simulink subsystem "FuelCellCore"  (R2025b)
settings: Solver=VariableStepAuto  StartTime=0.0  StopTime=10.0  RelTol=1e-3
undefined symbols (not defined in the file): PlntFcAuxPwrMap, PlntFcCurrBpt, PlntFcH2FlwMap, PlntFcHeatFlwMap, PlntFcTempBpt, PlntFcVoltageMap
settings Model: ModifiedByFormat=The MathWorks, Inc.  Creator=The MathWorks, Inc.  LastModifiedBy=The MathWorks, Inc.
settings SolverCC: MaxZcPerStep=1.0
settings OptimizationCC: ReuseModelBlockBuffer=off
settings DebuggingCC: UnconnectedInputMsg=warning  UnconnectedOutputMsg=warning  UnconnectedLineMsg=warning  SubsystemReferenceDiagnosticForUnitTest=warning
settings ModelReferenceCC: EnableRefExpFcnMdlSchedulingChecks=on
settings RTWCC: GPUComputeCapability=3.5  DLArmComputeVersion=19.05

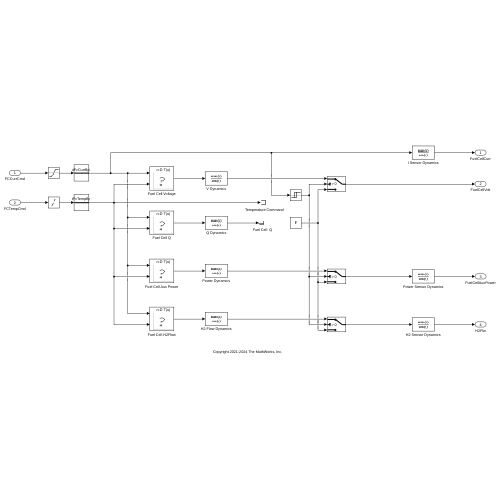
[thumbnail: Simulink's stored preview of the top-level diagram]
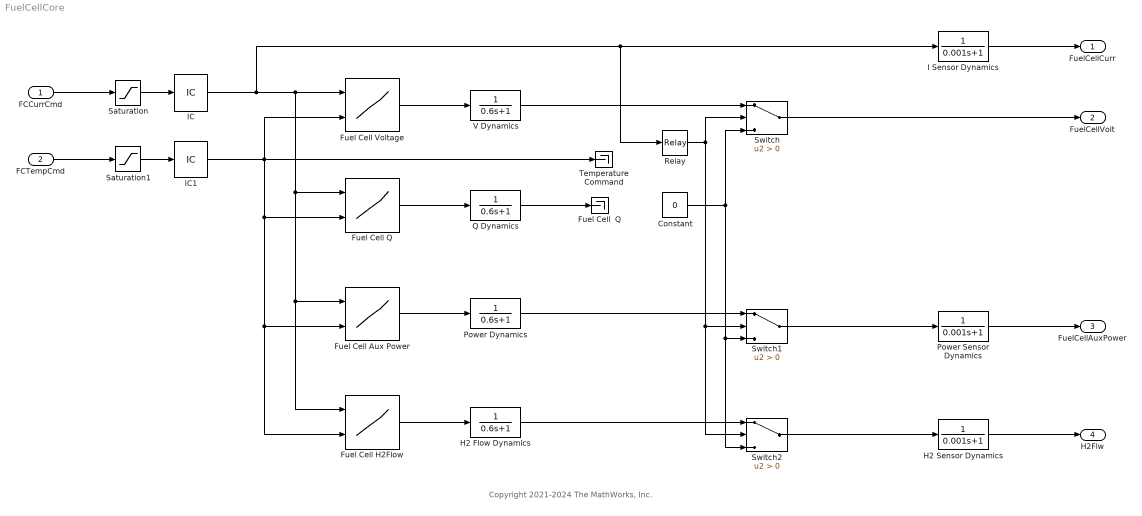
== system FuelCellCore ==
  note: Copyright 2021-2024 The MathWorks, Inc.
  FCCurrCmd : Inport
  FCTempCmd : Inport  Port=2
  Constant : Constant  Value=0
  Fuel Cell  Q : Terminator
  Fuel Cell Aux Power : Lookup_n-D  BreakpointsForDimension1=PlntFcCurrBpt  BreakpointsForDimension2=PlntFcTempBpt  Table=PlntFcAuxPwrMap  ExtrapMethod=Clip  InternalRulePriority=Speed  RndMeth=Simplest
      settings: InputPortMap=u0,u1
  Fuel Cell H2Flow : Lookup_n-D  BreakpointsForDimension1=PlntFcCurrBpt  BreakpointsForDimension2=PlntFcTempBpt  Table=PlntFcH2FlwMap  ExtrapMethod=Clip  InternalRulePriority=Speed  RndMeth=Simplest
      settings: InputPortMap=u0,u1
  Fuel Cell Q : Lookup_n-D  BreakpointsForDimension1=PlntFcCurrBpt  BreakpointsForDimension2=PlntFcTempBpt  Table=PlntFcHeatFlwMap  ExtrapMethod=Clip  InternalRulePriority=Speed  RndMeth=Simplest
      settings: InputPortMap=u0,u1
  Fuel Cell Voltage : Lookup_n-D  BreakpointsForDimension1=PlntFcCurrBpt  BreakpointsForDimension2=PlntFcTempBpt  Table=PlntFcVoltageMap  ExtrapMethod=Clip  InternalRulePriority=Speed  RndMeth=Simplest
      settings: InputPortMap=u0,u1
  H2 Flow Dynamics : TransferFcn  Denominator=[0.6 1]
  H2 Sensor Dynamics : TransferFcn  Denominator=[0.001 1]
  I Sensor Dynamics : TransferFcn  Denominator=[0.001 1]
  IC : InitialCondition  Value=PlntFcCurrBpt(1)
  IC1 : InitialCondition  Value=PlntFcTempBpt(1)
  Power Dynamics : TransferFcn  Denominator=[0.6 1]
  Power Sensor Dynamics : TransferFcn  Denominator=[0.001 1]
  Q Dynamics : TransferFcn  Denominator=[0.6 1]
  Relay : Relay
  Saturation : Saturate  UpperLimit=max(PlntFcCurrBpt)  LowerLimit=0  ZeroCross=off
  Saturation1 : Saturate  UpperLimit=max(PlntFcTempBpt)  LowerLimit=0  ZeroCross=off
  Switch : Switch  Criteria=u2 > Threshold  ZeroCross=off  SaturateOnIntegerOverflow=off  InputSameDT=off
  Switch1 : Switch  Criteria=u2 > Threshold  ZeroCross=off  SaturateOnIntegerOverflow=off  InputSameDT=off
  Switch2 : Switch  Criteria=u2 > Threshold  ZeroCross=off  SaturateOnIntegerOverflow=off  InputSameDT=off
  Temperature Command : Terminator
  V Dynamics : TransferFcn  Denominator=[0.6 1]
  FuelCellCurr : Outport
  FuelCellVolt : Outport  Port=2
  FuelCellAuxPower : Outport  Port=3
  H2Flw : Outport  Port=4
  wires:
  Q Dynamics/1 -> Fuel Cell  Q/1
  Saturation1/1 -> IC1/1
  H2 Sensor Dynamics/1 -> H2Flw/1
  FCCurrCmd/1 -> Saturation/1
  I Sensor Dynamics/1 -> FuelCellCurr/1
  FCTempCmd/1 -> Saturation1/1
  Power Dynamics/1 -> Switch1/1
  Fuel Cell Q/1 -> Q Dynamics/1
  Power Sensor Dynamics/1 -> FuelCellAuxPower/1
  Fuel Cell Voltage/1 -> V Dynamics/1
  Fuel Cell H2Flow/1 -> H2 Flow Dynamics/1
  V Dynamics/1 -> Switch/1
  Saturation/1 -> IC/1
  H2 Flow Dynamics/1 -> Switch2/1
  Fuel Cell Aux Power/1 -> Power Dynamics/1
  IC/1 -> Fuel Cell Voltage/1, Fuel Cell Q/1, Fuel Cell Aux Power/1, Fuel Cell H2Flow/1, I Sensor Dynamics/1, Relay/1
  IC1/1 -> Temperature Command/1, Fuel Cell Q/2, Fuel Cell Aux Power/2, Fuel Cell H2Flow/2, Fuel Cell Voltage/2
  Relay/1 -> Switch2/2, Switch1/2, Switch/2
  Constant/1 -> Switch1/3, Switch2/3, Switch/3
  Switch/1 -> FuelCellVolt/1
  Switch1/1 -> Power Sensor Dynamics/1
  Switch2/1 -> H2 Sensor Dynamics/1
